simulink model "Logical_Operators"  (R2024b)
settings: Solver=VariableStepAuto  StartTime=0.0  StopTime=10.0  RelTol=1e-3
libraries: simulink x4
settings Model: Creator=Ahmad  LastModifiedBy=Ahmad

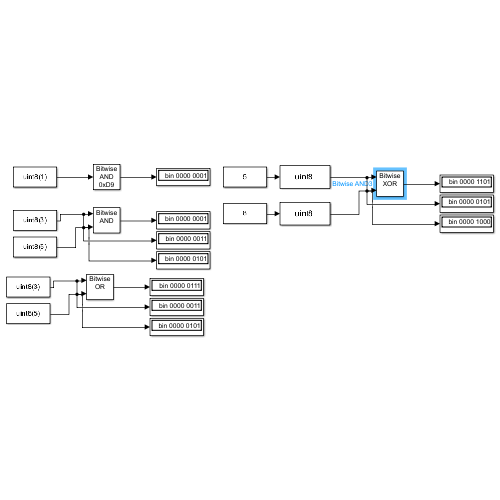
[thumbnail: Simulink's stored preview of the top-level diagram]
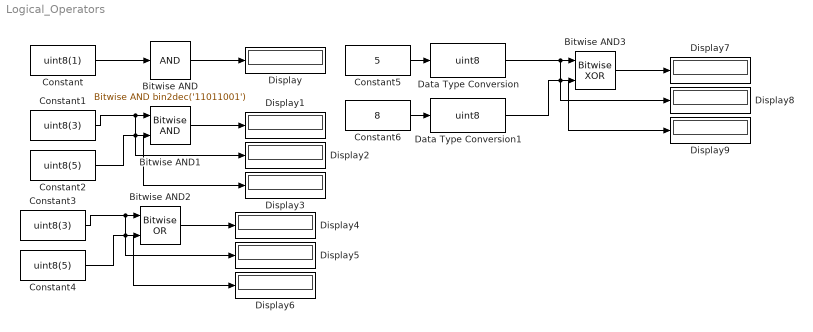
== system Logical_Operators ==
  Bitwise AND : simulink/Logic and Bit Operations/Bitwise Operator  logicop=AND  UseBitMask=on  BitMask=bin2dec('11011001')  BitMaskRealWorld=Stored Integer
      settings: LibrarySourceBlock=|
      | simulink/Quick Insert/Logic and Bit
      | Operations/Bitwise AND
  Bitwise AND1 : simulink/Logic and Bit Operations/Bitwise Operator  logicop=AND  UseBitMask=off  NumInputPorts=2  BitMask=bin2dec('11011001')  BitMaskRealWorld=Stored Integer
      settings: LibrarySourceBlock=|
      | simulink/Quick Insert/Logic and Bit
      | Operations/Bitwise AND
  Bitwise AND2 : simulink/Logic and Bit Operations/Bitwise Operator  logicop=OR  UseBitMask=off  NumInputPorts=2  BitMask=bin2dec('11011001')  BitMaskRealWorld=Stored Integer
      settings: LibrarySourceBlock=|
      | simulink/Quick Insert/Logic and Bit
      | Operations/Bitwise AND
  Bitwise AND3 : simulink/Logic and Bit Operations/Bitwise Operator  logicop=XOR  UseBitMask=off  NumInputPorts=2  BitMask=bin2dec('11011001')  BitMaskRealWorld=Stored Integer
      settings: LibrarySourceBlock=|
      | simulink/Quick Insert/Logic and Bit
      | Operations/Bitwise AND
  Constant : Constant  Value=uint8(1)
  Constant1 : Constant  Value=uint8(3)
  Constant2 : Constant  Value=uint8(5)
  Constant3 : Constant  Value=uint8(3)
  Constant4 : Constant  Value=uint8(5)
  Constant5 : Constant  Value=5
  Constant6 : Constant  Value=8
  Data Type Conversion : DataTypeConversion  OutDataTypeStr=uint8  SaturateOnIntegerOverflow=off  RndMeth=Floor
  Data Type Conversion1 : DataTypeConversion  OutDataTypeStr=uint8  SaturateOnIntegerOverflow=off  RndMeth=Floor
  Display{,1..9} (10 alike) : Display
      settings: Format=binary (Stored Integer)
  wires:
  Bitwise AND/1 -> Display/1
  Constant/1 -> Bitwise AND/1
  Constant1/1 -> Display2/1, Bitwise AND1/1
  Bitwise AND1/1 -> Display1/1
  Constant2/1 -> Display3/1, Bitwise AND1/2
  Bitwise AND2/1 -> Display4/1
  Constant4/1 -> Display6/1, Bitwise AND2/2
  Constant3/1 -> Display5/1, Bitwise AND2/1
  Bitwise AND3/1 -> Display7/1
  Data Type Conversion1/1 -> Display9/1, Bitwise AND3/2
  Data Type Conversion/1 -> Display8/1, Bitwise AND3/1
  Constant5/1 -> Data Type Conversion/1
  Constant6/1 -> Data Type Conversion1/1
